simulink model "simpleLLS"  (Simulink 4.00)
settings: Solver=ode45  StartTime=0.0  StopTime=2.0  RelTol=1e-5  AbsTol=1e-5
settings Model: LastModifiedBy=hyzheng

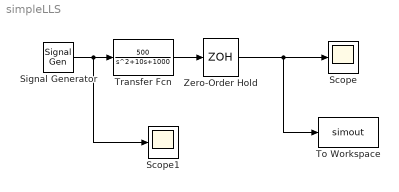
== system simpleLLS ==
  Scope : Scope
      settings: TimeRange=auto  YMin=-5  YMax=5  SaveToWorkspace=off  SaveName=ScopeData  LimitDataPoints=on  MaxDataPoints=5000
  Scope1 : Scope
      settings: TimeRange=auto  YMin=-5  YMax=5  SaveToWorkspace=off  LimitDataPoints=on  MaxDataPoints=5000
  Signal Generator : SignalGenerator  WaveForm=square  Amplitude=-2  Frequency=0.5  Units=Hertz
  To Workspace : ToWorkspace  VariableName=simout  SampleTime=-1  SaveFormat=Array
  Transfer Fcn : TransferFcn  Numerator=[500]  Denominator=[1 10 1000]  AbsoluteTolerance=1e-5  Realization=auto
  Zero-Order Hold : ZeroOrderHold  SampleTime=0.1
  wires:
  Signal Generator/1 -> Transfer Fcn/1, Scope1/1
  Transfer Fcn/1 -> Zero-Order Hold/1
  Zero-Order Hold/1 -> Scope/1, To Workspace/1
